simulink model "ES101A_DiagcMgr"  (R2013b)
settings: Solver=ode45  StartTime=0.0  StopTime=0.44  RelTol=1e-3
values from neighbouring files (symbols this model uses):
  BrdgVltg = DataDict.IpSignal    [ES101A_DiagcMgr_DataDict.m]
  DEM_CLEAR_PENDING = DataDict.Constant    [ES101A_DiagcMgr_DataDict.m]
  DEM_DTC_GROUP_ALL_DTCS = DataDict.Constant    [ES101A_DiagcMgr_DataDict.m]
  DFTAGICNTR_CNT_U08 = DataDict.Constant    [ES101A_DiagcMgr_DataDict.m]
  DIAGCMGR_NTCINFOSTSTESTFAILD_CNT_U08 = DataDict.Constant    [ES101A_DiagcMgrProxyX_DataDict.m]    (also in ES101A_DiagcMgr_DataDict.m)
  DIAGCMGR_NTCINFOSTSTESTFAILDTHISIGNCYC_CNT_U08 = DataDict.Constant    [ES101A_DiagcMgr_DataDict.m]
  DIAGCMGR_NTCINFOSTSTESTNOTCMPLTHISIGNCYC_CNT_U08 = DataDict.Constant    [ES101A_DiagcMgrProxyX_DataDict.m]    (also in ES101A_DiagcMgr_DataDict.m)
  DiagcMgrFltResp = DataDict.Calibration    [ES101A_DiagcMgrProxyX_DataDict.m]    (also in ES101A_DiagcMgr_DataDict.m)
  DiagcMgrNtcFltAry = DataDict.NVM    [ES101A_DiagcMgr_DataDict.m]
  DIAGCSTSCTRLDSHTDWNFLTPRSNT_CNT_U16 = DataDict.Constant    [ES101A_DiagcMgr_DataDict.m]
  DIAGCSTSDFTHWAG_CNT_U16 = DataDict.Constant    [ES101A_DiagcMgr_DataDict.m]
  DIAGCSTSDFTHWAGSERLCOMEXPRTVAL_CNT_U16 = DataDict.Constant    [ES101A_DiagcMgr_DataDict.m]
  DIAGCSTSDFTVEHSPD_CNT_U16 = DataDict.Constant    [ES101A_DiagcMgr_DataDict.m]
  DIAGCSTSININVAL_CNT_U16 = DataDict.Constant    [ES101A_DiagcMgrProxyX_DataDict.m]    (also in ES101A_DiagcMgr_DataDict.m)
  DIAGCSTSIVTR1INACTV_CNT_U16 = DataDict.Constant    [ES101A_DiagcMgr_DataDict.m]
  DIAGCSTSIVTR2INACTV_CNT_U16 = DataDict.Constant    [ES101A_DiagcMgr_DataDict.m]
  DIAGCSTSLIMDTPRFMNC_CNT_U16 = DataDict.Constant    [ES101A_DiagcMgr_DataDict.m]
  DIAGCSTSRAMPTOZEROFLTPRSNT_CNT_U16 = DataDict.Constant    [ES101A_DiagcMgr_DataDict.m]
  DIAGCSTSWHLIMBREJCTNDI_CNT_U16 = DataDict.Constant    [ES101A_DiagcMgr_DataDict.m]
  DTCIDXSTSFAIL_CNT_U08 = DataDict.Constant    [ES101A_DiagcMgr_DataDict.m]
  DTCIDXSTSNONTC_CNT_U08 = DataDict.Constant    [ES101A_DiagcMgr_DataDict.m]
  DTCIDXSTSNORES_CNT_U08 = DataDict.Constant    [ES101A_DiagcMgr_DataDict.m]
  DTCIDXSTSPASS_CNT_U08 = DataDict.Constant    [ES101A_DiagcMgr_DataDict.m]
  DTCIDXSTSUPDCFMD_CNT_U08 = DataDict.Constant    [ES101A_DiagcMgr_DataDict.m]
  ELECGLBPRM_IVTRCNT_CNT_U08 = DataDict.ConfigParam    [ES101A_DiagcMgrProxyX_DataDict.m]    (also in ES101A_DiagcMgr_DataDict.m)
  FLTINJ_DIAGCMGR_DIAGCSTSIVTR1INACTV = DataDict.Constant    [ES101A_DiagcMgr_DataDict.m]
  FLTINJ_DIAGCMGR_DIAGCSTSIVTR2INACTV = DataDict.Constant    [ES101A_DiagcMgr_DataDict.m]
  HwTq = DataDict.IpSignal    [ES101A_DiagcMgr_DataDict.m]
  IgnCntr = DataDict.IpSignal    [ES101A_DiagcMgr_DataDict.m]
  MAXDEBCNTRVAL_CNT_S16 = DataDict.Constant    [ES101A_DiagcMgr_DataDict.m]
  MAXRAMPRATE_ULSPERSEC_F32 = DataDict.Constant    [ES101A_DiagcMgrProxyX_DataDict.m]    (also in ES101A_DiagcMgr_DataDict.m)
  MINDEBCNTRVAL_CNT_S16 = DataDict.Constant    [ES101A_DiagcMgr_DataDict.m]
  MINRAMPRATE_ULSPERSEC_F32 = DataDict.Constant    [ES101A_DiagcMgrProxyX_DataDict.m]    (also in ES101A_DiagcMgr_DataDict.m)
  SCAMOTTQCMDTOONE_ULS_F32 = DataDict.Constant    [ES101A_DiagcMgrProxyX_DataDict.m]    (also in ES101A_DiagcMgr_DataDict.m)
  SCAMOTTQCMDTOZERO_ULS_F32 = DataDict.Constant    [ES101A_DiagcMgrProxyX_DataDict.m]    (also in ES101A_DiagcMgr_DataDict.m)
  SysSt = DataDict.IpSignal    [ES101A_DiagcMgr_DataDict.m]
  VehSpd = DataDict.IpSignal    [ES101A_DiagcMgr_DataDict.m]
undefined symbols (not defined in the file or in its folder): ActvMotTqCmdSca, ActvRampRate, AgiCntr, Dem_DTCFormatType, Dem_DTCOriginType, Dem_EventStatusType, DiagcData, DiagcMgrNtcMap, DiagcSts, DtcEnaMask, EcuT, HistNtcFltAry, MicroDiagcData, MotTq, NtcNr, NtcNrWithResd1, NtcStInfo, ProxySetNtcData, Sts, SysSt1, TOTNROFDTC_CNT_U08
libraries: simulink x149, FloatToFixd x5, NxtrNvM x3
(part 10 of 13)

== system ES101A_DiagcMgr/DiagcMgr/SetNtcStsCore/NtcNr is Valid/Diagnostics Not Inhibited/NtcEnabled/NTCSTS_PREFAILD/Update NtcInfoSts, DebCntr and Process RampRate/DebCntr = MAXDEBCNTRVAL_CNT_S16/Update NtcSts and DebCntr ==
  NtcInfo_ArgIn : Inport
  NtcStInfo_ArgIn : Inport  Port=2
  Bus Assignment1 : BusAssignment  AssignedSignals=Sts,NtcStInfo,AgiCntr
  Bus Selector : BusSelector  OutputSignals=Sts,NtcStInfo
  Clear: DIAGCMGR_NTCINFOSTSTESTNOTCMPLTHISIGNCYC_CNT_U08 : Subsystem
  Constant : Constant  Value=MAXDEBCNTRVAL_CNT_S16
  Constant1 : Constant  Value=DIAGCMGR_NTCINFOSTSTESTNOTCMPLTHISIGNCYC_CNT_U08
  Constant2 : Constant  Value=0  OutDataTypeStr=uint8
  Copyright1 : Subsystem  Description=|  mask(Copyright Information){none=on}
      | Copyright info block.                                               
      |                                                                     
      | Place copyright information at the top of every subsystem in design.
      mask prompts: none "No parameters"
      mask help: Place copyright information at the top of every subsystem in design.
      mask Display:
      | NxtrConf = 'Nexteer Confidential';
      | 
      | sys = bdroot; %handle for the current model ("system")
      | first = get_param(sys,'Created');
      | if(isempty(first))
      |     first = datestr(now,'yyyy');
      | else
      |     first = first(end-3:end);  %year is last four digits
      | end
      | 
      | last = get_param(sys,'LastModifiedDate');
      | if isempty(last)
      |     last = datestr(now,'yyyy');
      | else
      |     last = last(end-3:end);
      | end
      | 
      | if strcmp(first,last)
      |     fprintf('%s\nCopyright  %s Nexteer',NxtrConf,first);
      | else
      |     fprintf('%s\n%s%s-%s Nexteer',NxtrConf,char(169),first,last);
      | end
  Set Bit: DIAGCMGR_NTCINFOCFMDNTC_CNT_U08 : simulink/Logic and Bit Operations/Bitwise Operator  logicop=OR  UseBitMask=on  BitMask=DIAGCMGR_NTCINFOCFMDNTC_CNT_U08  BitMaskRealWorld=Stored Integer
  Set Bits: DIAGCMGR_NTCINFOSTSTESTFAILDTHISIGNCYC_CNT_U08 : simulink/Logic and Bit Operations/Bitwise Operator  logicop=OR  UseBitMask=on  BitMask=DIAGCMGR_NTCINFOSTSTESTFAILDTHISIGNCYC_CNT_U08  BitMaskRealWorld=Stored Integer
  Set Bits: DIAGCMGR_NTCINFOSTSTESTFAILD_CNT_U08 : simulink/Logic and Bit Operations/Bitwise Operator  logicop=OR  UseBitMask=on  BitMask=DIAGCMGR_NTCINFOSTSTESTFAILD_CNT_U08  BitMaskRealWorld=Stored Integer
  Update NtcStInfo : simulink/Logic and Bit Operations/Bitwise Operator  logicop=OR  UseBitMask=off  NumInputPorts=2  BitMask=bin2dec('11')  BitMaskRealWorld=Stored Integer
  NtcInfo_ArgOut : Outport
  NtcInfoDebCntr_ArgOut : Outport  Port=2
  wires:
  NtcInfo_ArgIn/1 -> Bus Assignment1/1, Bus Selector/1
  Constant/1 -> NtcInfoDebCntr_ArgOut/1
  Bus Assignment1/1 -> NtcInfo_ArgOut/1
  Clear: DIAGCMGR_NTCINFOSTSTESTNOTCMPLTHISIGNCYC_CNT_U08/1(Out1) -> Bus Assignment1/2
  NtcStInfo_ArgIn/1 -> Update NtcStInfo/2
  Update NtcStInfo/1 -> Bus Assignment1/3
  Bus Selector/2 -> Update NtcStInfo/1  "<NtcStInfo>"
  Constant2/1 -> Bus Assignment1/4
  Constant1/1 -> Clear: DIAGCMGR_NTCINFOSTSTESTNOTCMPLTHISIGNCYC_CNT_U08/2(In1)
  Set Bits: DIAGCMGR_NTCINFOSTSTESTFAILD_CNT_U08/1 -> Set Bits: DIAGCMGR_NTCINFOSTSTESTFAILDTHISIGNCYC_CNT_U08/1
  Set Bits: DIAGCMGR_NTCINFOSTSTESTFAILDTHISIGNCYC_CNT_U08/1 -> Set Bit: DIAGCMGR_NTCINFOCFMDNTC_CNT_U08/1
  Set Bit: DIAGCMGR_NTCINFOCFMDNTC_CNT_U08/1 -> Clear: DIAGCMGR_NTCINFOSTSTESTNOTCMPLTHISIGNCYC_CNT_U08/1(In2)
  Bus Selector/1 -> Set Bits: DIAGCMGR_NTCINFOSTSTESTFAILD_CNT_U08/1  "<Sts>"

== system ES101A_DiagcMgr/DiagcMgr/SetNtcStsCore/NtcNr is Valid/Diagnostics Not Inhibited/NtcEnabled/NTCSTS_PREPASSD/Update NtcInfoSts/Do Nothing/CopyRight2 ==

== system ES101A_DiagcMgr/DiagcMgr/SetNtcStsCore/NtcNr is Valid/Diagnostics Not Inhibited/NtcEnabled/NTCSTS_PREPASSD/Update NtcInfoSts/Update NTC Info's Status Byte & Update the NTC Fault Array/CopyRight2 ==

== system ES101A_DiagcMgr/DiagcMgr/SetNtcStsCore/NtcNr is Valid/Diagnostics Not Inhibited/NtcEnabled/NTCSTS_PREPASSD/Update NtcInfoSts/Update NTC Info's Status Byte & Update the NTC Fault Array/Decrement Counter ==
  "NtcInfo_ArgIn " : Inport
  DebStep_ArgIn : Inport  Port=2
  NtcInfoDebCntr_ArgIn : Inport  Port=3
  Constant : Constant  Value=MINDEBCNTRVAL_CNT_S16
  Copyright1 : Subsystem  Description=|  mask(Copyright Information){none=on}
      | Copyright info block.                                               
      |                                                                     
      | Place copyright information at the top of every subsystem in design.
      mask prompts: none "No parameters"
      mask help: Place copyright information at the top of every subsystem in design.
      mask Display:
      | NxtrConf = 'Nexteer Confidential';
      | 
      | sys = bdroot; %handle for the current model ("system")
      | first = get_param(sys,'Created');
      | if(isempty(first))
      |     first = datestr(now,'yyyy');
      | else
      |     first = first(end-3:end);  %year is last four digits
      | end
      | 
      | last = get_param(sys,'LastModifiedDate');
      | if isempty(last)
      |     last = datestr(now,'yyyy');
      | else
      |     last = last(end-3:end);
      | end
      | 
      | if strcmp(first,last)
      |     fprintf('%s\nCopyright  %s Nexteer',NxtrConf,first);
      | else
      |     fprintf('%s\n%s%s-%s Nexteer',NxtrConf,char(169),first,last);
      | end
  Deb Counter > MINDEBCNTRVAL_CNT_S16 : Subsystem  TreatAsAtomicUnit=on
  DebCntr = MINDEBCNTRVAL_CNT_S16 : Subsystem  TreatAsAtomicUnit=on
  If1 : If  NumInputs=2  IfExpression="u1 <=  u2"
  Merge1 : Merge
  Sub1 : Sum  SaturateOnIntegerOverflow=on
  NtcInfo_ArgOut : Outport
  NtcInfoDebCntr_ArgOut : Outport  Port=2
  wires:
  If1/1 -> DebCntr = MINDEBCNTRVAL_CNT_S16/Action
  If1/2 -> Deb Counter > MINDEBCNTRVAL_CNT_S16/Action
  DebStep_ArgIn/1 -> Sub1/1, Deb Counter > MINDEBCNTRVAL_CNT_S16/1(DebStep)
  "NtcInfo_ArgIn "/1 -> DebCntr = MINDEBCNTRVAL_CNT_S16/1(NtcInfo_ArgIn)
  Constant/1 -> Sub1/2
  Sub1/1 -> If1/2
  Deb Counter > MINDEBCNTRVAL_CNT_S16/1(NtcInfoDebCntr_ArgOut) -> Merge1/2
  DebCntr = MINDEBCNTRVAL_CNT_S16/1(NtcInfo_ArgOut) -> NtcInfo_ArgOut/1
  DebCntr = MINDEBCNTRVAL_CNT_S16/2(NtcInfoDebCntr_ArgOut) -> Merge1/1
  Merge1/1 -> NtcInfoDebCntr_ArgOut/1
  NtcInfoDebCntr_ArgIn/1 -> Deb Counter > MINDEBCNTRVAL_CNT_S16/2(NtcInfoDebCntr_ArgIn), If1/1

== system ES101A_DiagcMgr/DiagcMgr/DiagcMgrPer2/Normal Periodic Processing/For All DTCs/For Each DTC/Check If DTC Status has Changed/DTC Status Changed OR DTC Update NOT Confirmed/Update DTC Status/Dtc Status is Failed/CopyRight2 ==

== system ES101A_DiagcMgr/DiagcMgr/DiagcMgrPer2/Normal Periodic Processing/For All DTCs/For Each DTC/Check If DTC Status has Changed/DTC Status Changed OR DTC Update NOT Confirmed/Update DTC Status/Dtc Status is Failed/Dem_SetEventStatus ==
  EventId : Inport
  EventStatus : Inport  Port=2
  CopyRight2 : Subsystem  Description=|  mask(Copyright Information){none=on}
      | Copyright info block.                                               
      |                                                                     
      | Place copyright information at the top of every subsystem in design.
      mask prompts: none "No parameters"
      mask help: Place copyright information at the top of every subsystem in design.
      mask Display:
      | NxtrConf = 'Nexteer Confidential';
      | 
      | sys = bdroot; %handle for the current model ("system")
      | first = get_param(sys,'Created');
      | first = first(end-3:end);  %year is last four digits
      | 
      | last = get_param(sys,'LastModifiedDate');
      | if isempty(last)
      |     last = datestr(now,'yyyy');
      | else
      |     last = last(end-3:end);
      | end
      | 
      | if strcmp(first,last)
      |     fprintf('%s -- Copyright %s Nexteer',NxtrConf,first)
      | else
      |     fprintf('%s -- %s%s- %s Nexteer',NxtrConf,char(169),first,last)
      | end
  Ground : Ground
  Terminator : Terminator
  Terminator1 : Terminator
  Dem_SetEventStatus_StdRtn : Outport
  wires:
  Ground/1 -> Dem_SetEventStatus_StdRtn/1
  EventStatus/1 -> Terminator1/1
  EventId/1 -> Terminator/1

== system ES101A_DiagcMgr/DiagcMgr/DiagcMgrPer2/Normal Periodic Processing/For All DTCs/For Each DTC/Check If DTC Status has Changed/DTC Status Changed OR DTC Update NOT Confirmed/Update DTC Status/Dtc Status is Failed/Update 'DTC Index Update Confirmed' Bit ==
  Dem_SetEventStatus_StdRtn : Inport
  DtcIdxPrevSts : Inport  Port=2
  DtcIdx : Inport  Port=3
  CopyRight2 : Subsystem  Description=|  mask(Copyright Information){none=on}
      | Copyright info block.                                               
      |                                                                     
      | Place copyright information at the top of every subsystem in design.
      mask prompts: none "No parameters"
      mask help: Place copyright information at the top of every subsystem in design.
      mask Display:
      | NxtrConf = 'Nexteer Confidential';
      | 
      | sys = bdroot; %handle for the current model ("system")
      | first = get_param(sys,'Created');
      | first = first(end-3:end);  %year is last four digits
      | 
      | last = get_param(sys,'LastModifiedDate');
      | if isempty(last)
      |     last = datestr(now,'yyyy');
      | else
      |     last = last(end-3:end);
      | end
      | 
      | if strcmp(first,last)
      |     fprintf('%s -- Copyright %s Nexteer',NxtrConf,first)
      | else
      |     fprintf('%s -- %s%s- %s Nexteer',NxtrConf,char(169),first,last)
      | end
  If : If  IfExpression=u1 == 0  ShowElse=off
  StdRtn is E_OK : Subsystem  TreatAsAtomicUnit=on
  wires:
  DtcIdxPrevSts/1 -> StdRtn is E_OK/2(DtcIdxPrevSts)
  DtcIdx/1 -> StdRtn is E_OK/1(DtcIdx)
  If/1 -> StdRtn is E_OK/Action
  Dem_SetEventStatus_StdRtn/1 -> If/1

== system ES101A_DiagcMgr/DiagcMgr/DiagcMgrPer2/Normal Periodic Processing/For All DTCs/For Each DTC/Check If DTC Status has Changed/DTC Status Changed OR DTC Update NOT Confirmed/Update DTC Status/Dtc Status is No Result or No Ntc/CopyRight2 ==

== system ES101A_DiagcMgr/DiagcMgr/DiagcMgrPer2/Normal Periodic Processing/For All DTCs/For Each DTC/Check If DTC Status has Changed/DTC Status Changed OR DTC Update NOT Confirmed/Update DTC Status/Dtc Status is No Result or No Ntc/Set Bit 7 (DTC Update Confirmed) ==
  In1 : Inport
  Bitwise Operator1 : simulink/Logic and Bit Operations/Bitwise Operator  logicop=OR  UseBitMask=off  NumInputPorts=2  BitMask=bin2dec('11011001')  BitMaskRealWorld=Stored Integer
  CopyRight2 : Subsystem  Description=|  mask(Copyright Information){none=on}
      | Copyright info block.                                               
      |                                                                     
      | Place copyright information at the top of every subsystem in design.
      mask prompts: none "No parameters"
      mask help: Place copyright information at the top of every subsystem in design.
      mask Display:
      | NxtrConf = 'Nexteer Confidential';
      | 
      | sys = bdroot; %handle for the current model ("system")
      | first = get_param(sys,'Created');
      | first = first(end-3:end);  %year is last four digits
      | 
      | last = get_param(sys,'LastModifiedDate');
      | if isempty(last)
      |     last = datestr(now,'yyyy');
      | else
      |     last = last(end-3:end);
      | end
      | 
      | if strcmp(first,last)
      |     fprintf('%s -- Copyright %s Nexteer',NxtrConf,first)
      | else
      |     fprintf('%s -- %s%s- %s Nexteer',NxtrConf,char(169),first,last)
      | end
  DTC Previous Status Bit 7 : Constant  Value=DTCIDXSTSUPDCFMD_CNT_U08
  Out1 : Outport
  wires:
  DTC Previous Status Bit 7/1 -> Bitwise Operator1/2
  In1/1 -> Bitwise Operator1/1
  Bitwise Operator1/1 -> Out1/1

== system ES101A_DiagcMgr/DiagcMgr/DiagcMgrPer2/Normal Periodic Processing/For All DTCs/For Each DTC/Check If DTC Status has Changed/DTC Status Changed OR DTC Update NOT Confirmed/Update DTC Status/Dtc Status is Passed/CopyRight2 ==

== system ES101A_DiagcMgr/DiagcMgr/DiagcMgrPer2/Normal Periodic Processing/For All DTCs/For Each DTC/Check If DTC Status has Changed/DTC Status Changed OR DTC Update NOT Confirmed/Update DTC Status/Dtc Status is Passed/Dem_SetEventStatus ==
  EventId : Inport
  EventStatus : Inport  Port=2
  CopyRight2 : Subsystem  Description=|  mask(Copyright Information){none=on}
      | Copyright info block.                                               
      |                                                                     
      | Place copyright information at the top of every subsystem in design.
      mask prompts: none "No parameters"
      mask help: Place copyright information at the top of every subsystem in design.
      mask Display:
      | NxtrConf = 'Nexteer Confidential';
      | 
      | sys = bdroot; %handle for the current model ("system")
      | first = get_param(sys,'Created');
      | first = first(end-3:end);  %year is last four digits
      | 
      | last = get_param(sys,'LastModifiedDate');
      | if isempty(last)
      |     last = datestr(now,'yyyy');
      | else
      |     last = last(end-3:end);
      | end
      | 
      | if strcmp(first,last)
      |     fprintf('%s -- Copyright %s Nexteer',NxtrConf,first)
      | else
      |     fprintf('%s -- %s%s- %s Nexteer',NxtrConf,char(169),first,last)
      | end
  Ground : Ground
  Terminator : Terminator
  Terminator1 : Terminator
  Dem_SetEventStatus_StdRtn : Outport
  wires:
  EventId/1 -> Terminator/1
  EventStatus/1 -> Terminator1/1
  Ground/1 -> Dem_SetEventStatus_StdRtn/1

== system ES101A_DiagcMgr/DiagcMgr/DiagcMgrPer2/Normal Periodic Processing/For All DTCs/For Each DTC/Check If DTC Status has Changed/DTC Status Changed OR DTC Update NOT Confirmed/Update DTC Status/Dtc Status is Passed/Update 'DTC Index Update Confirmed' Bit ==
  Dem_SetEventStatus_StdRtn : Inport
  DtcIdxPrevSts : Inport  Port=2
  DtcIdx : Inport  Port=3
  CopyRight2 : Subsystem  Description=|  mask(Copyright Information){none=on}
      | Copyright info block.                                               
      |                                                                     
      | Place copyright information at the top of every subsystem in design.
      mask prompts: none "No parameters"
      mask help: Place copyright information at the top of every subsystem in design.
      mask Display:
      | NxtrConf = 'Nexteer Confidential';
      | 
      | sys = bdroot; %handle for the current model ("system")
      | first = get_param(sys,'Created');
      | first = first(end-3:end);  %year is last four digits
      | 
      | last = get_param(sys,'LastModifiedDate');
      | if isempty(last)
      |     last = datestr(now,'yyyy');
      | else
      |     last = last(end-3:end);
      | end
      | 
      | if strcmp(first,last)
      |     fprintf('%s -- Copyright %s Nexteer',NxtrConf,first)
      | else
      |     fprintf('%s -- %s%s- %s Nexteer',NxtrConf,char(169),first,last)
      | end
  If : If  IfExpression=u1 == 0  ShowElse=off
  StdRtn is E_OK : Subsystem  TreatAsAtomicUnit=on
  wires:
  Dem_SetEventStatus_StdRtn/1 -> If/1
  If/1 -> StdRtn is E_OK/Action
  DtcIdx/1 -> StdRtn is E_OK/1(DtcIdx)
  DtcIdxPrevSts/1 -> StdRtn is E_OK/2(DtcIdxPrevSts)

== system ES101A_DiagcMgr/DiagcMgr/SetNtcStsCore/NtcNr is Valid/Diagnostics Not Inhibited/NtcEnabled/NTCSTS_FAILD/Update ISO Bits, Parameter Byte and AgiCntr /ProcessRampResponse and DiagcSts/ControlledShutdown Fault/Atomic Section2 ==
  TmpDiagcSts : Inport
  DiagcData_ArgInOut : Inport  Port=2
  ProxySetNtcData_ArgInOut : Inport  Port=3
  Bitwise Operator : simulink/Logic and Bit Operations/Bitwise Operator  logicop=OR  UseBitMask=off  NumInputPorts=2  BitMask=bin2dec('11011001')  BitMaskRealWorld=Stored Integer
  Bitwise Operator1 : simulink/Logic and Bit Operations/Bitwise Operator  logicop=OR  UseBitMask=off  NumInputPorts=2  BitMask=bin2dec('11011001')  BitMaskRealWorld=Stored Integer
  Bus Creator2 : BusCreator  Inputs=2  OutDataTypeStr=Bus: DiagcData1  NonVirtualBus=on
  Bus Creator3 : BusCreator  Inputs=2  OutDataTypeStr=Bus: DiagcData1  NonVirtualBus=on
  Bus Selector : BusSelector  OutputSignals=DiagcSts,ActvMotTqCmdSca
  Bus Selector1 : BusSelector  OutputSignals=DiagcSts,ActvMotTqCmdSca
  CopyRight2 : Subsystem  Description=|  mask(Copyright Information){none=on}
      | Copyright info block.                                               
      |                                                                     
      | Place copyright information at the top of every subsystem in design.
      mask prompts: none "No parameters"
      mask help: Place copyright information at the top of every subsystem in design.
      mask Display:
      | NxtrConf = 'Nexteer Confidential';
      | 
      | sys = bdroot; %handle for the current model ("system")
      | first = get_param(sys,'Created');
      | first = first(end-3:end);  %year is last four digits
      | 
      | last = get_param(sys,'LastModifiedDate');
      | if isempty(last)
      |     last = datestr(now,'yyyy');
      | else
      |     last = last(end-3:end);
      | end
      | 
      | if strcmp(first,last)
      |     fprintf('%s -- Copyright %s Nexteer',NxtrConf,first)
      | else
      |     fprintf('%s -- %s%s- %s Nexteer',NxtrConf,char(169),first,last)
      | end
  If : If  NumInputs=2  IfExpression=u1 < u2  ShowElse=off
  If3 : If  NumInputs=2  IfExpression=u1 < u2  ShowElse=off
  Scale Motor Torque Command to Zero1 : Constant  Value=SCAMOTTQCMDTOZERO_ULS_F32  OutDataTypeStr=single
  Scale Motor Torque Command to Zero2 : Constant  Value=SCAMOTTQCMDTOZERO_ULS_F32  OutDataTypeStr=single
  Update Scale : Subsystem  TreatAsAtomicUnit=on
  Update Scale1 : Subsystem  TreatAsAtomicUnit=on
  DiagcData_ArgOut : Outport
  ProxySetNtcData_ArgOut : Outport  Port=2
  wires:
  Bus Selector/1 -> Bitwise Operator/1  "<DiagcSts>"
  If/1 -> Update Scale/Action
  Scale Motor Torque Command to Zero1/1 -> If/1
  TmpDiagcSts/1 -> Bitwise Operator1/2, Bitwise Operator/2
  Bus Selector1/1 -> Bitwise Operator1/1  "<DiagcSts>"
  If3/1 -> Update Scale1/Action
  Scale Motor Torque Command to Zero2/1 -> If3/1
  DiagcData_ArgInOut/1 -> Bus Selector/1
  ProxySetNtcData_ArgInOut/1 -> Bus Selector1/1
  Bus Selector/2 -> If/2  "<ActvMotTqCmdSca>"
  Bus Selector1/2 -> If3/2  "<ActvMotTqCmdSca>"
  Bitwise Operator/1 -> Bus Creator2/1
  Update Scale/1(DiagcMgrActvMotTqCmdSca) -> Bus Creator2/2
  Bus Creator2/1 -> DiagcData_ArgOut/1
  Bitwise Operator1/1 -> Bus Creator3/1
  Bus Creator3/1 -> ProxySetNtcData_ArgOut/1
  Update Scale1/1(ProxySetNtcMotTqCmdSca) -> Bus Creator3/2

== system ES101A_DiagcMgr/DiagcMgr/SetNtcStsCore/NtcNr is Valid/Diagnostics Not Inhibited/NtcEnabled/NTCSTS_FAILD/Update ISO Bits, Parameter Byte and AgiCntr /ProcessRampResponse and DiagcSts/ControlledShutdown Fault/CopyRight2 ==

== system ES101A_DiagcMgr/DiagcMgr/SetNtcStsCore/NtcNr is Valid/Diagnostics Not Inhibited/NtcEnabled/NTCSTS_FAILD/Update ISO Bits, Parameter Byte and AgiCntr /ProcessRampResponse and DiagcSts/InformationOnly Fault/Atomic Section2 ==
  DiagcData_ArgInOut : Inport
  ProxySetNtcData_ArgInOut : Inport  Port=2
  TmpDiagcSts : Inport  Port=3
  Bitwise Operator : simulink/Logic and Bit Operations/Bitwise Operator  logicop=OR  UseBitMask=off  NumInputPorts=2  BitMask=bin2dec('11011001')  BitMaskRealWorld=Stored Integer
  Bitwise Operator1 : simulink/Logic and Bit Operations/Bitwise Operator  logicop=OR  UseBitMask=off  NumInputPorts=2  BitMask=bin2dec('11011001')  BitMaskRealWorld=Stored Integer
  Bus Selector : BusSelector  OutputSignals=DiagcSts
  Bus Selector1 : BusSelector  OutputSignals=DiagcSts
  CopyRight2 : Subsystem  Description=|  mask(Copyright Information){none=on}
      | Copyright info block.                                               
      |                                                                     
      | Place copyright information at the top of every subsystem in design.
      mask prompts: none "No parameters"
      mask help: Place copyright information at the top of every subsystem in design.
      mask Display:
      | NxtrConf = 'Nexteer Confidential';
      | 
      | sys = bdroot; %handle for the current model ("system")
      | first = get_param(sys,'Created');
      | first = first(end-3:end);  %year is last four digits
      | 
      | last = get_param(sys,'LastModifiedDate');
      | if isempty(last)
      |     last = datestr(now,'yyyy');
      | else
      |     last = last(end-3:end);
      | end
      | 
      | if strcmp(first,last)
      |     fprintf('%s -- Copyright %s Nexteer',NxtrConf,first)
      | else
      |     fprintf('%s -- %s%s- %s Nexteer',NxtrConf,char(169),first,last)
      | end
  DiagcData_ArgOut : Outport
  ProxySetNtcData_ArgOut : Outport  Port=2
  wires:
  Bus Selector/1 -> Bitwise Operator/1  "<DiagcSts>"
  TmpDiagcSts/1 -> Bitwise Operator1/2, Bitwise Operator/2
  Bus Selector1/1 -> Bitwise Operator1/1  "<DiagcSts>"
  DiagcData_ArgInOut/1 -> Bus Selector/1
  ProxySetNtcData_ArgInOut/1 -> Bus Selector1/1
  Bitwise Operator/1 -> DiagcData_ArgOut/1
  Bitwise Operator1/1 -> ProxySetNtcData_ArgOut/1

== system ES101A_DiagcMgr/DiagcMgr/SetNtcStsCore/NtcNr is Valid/Diagnostics Not Inhibited/NtcEnabled/NTCSTS_FAILD/Update ISO Bits, Parameter Byte and AgiCntr /ProcessRampResponse and DiagcSts/InformationOnly Fault/CopyRight2 ==

== system ES101A_DiagcMgr/DiagcMgr/SetNtcStsCore/NtcNr is Valid/Diagnostics Not Inhibited/NtcEnabled/NTCSTS_FAILD/Update ISO Bits, Parameter Byte and AgiCntr /ProcessRampResponse and DiagcSts/ProcessDiagcSts/CopyRight2 ==

== system ES101A_DiagcMgr/DiagcMgr/SetNtcStsCore/NtcNr is Valid/Diagnostics Not Inhibited/NtcEnabled/NTCSTS_FAILD/Update ISO Bits, Parameter Byte and AgiCntr /ProcessRampResponse and DiagcSts/ProcessDiagcSts/If Action Subsystem ==
  Action Port : ActionPort
  Constant1 : Constant  Value=DIAGCSTSLIMDTPRFMNC_CNT_U16
  Out1 : Outport
  wires:
  Constant1/1 -> Out1/1

== system ES101A_DiagcMgr/DiagcMgr/SetNtcStsCore/NtcNr is Valid/Diagnostics Not Inhibited/NtcEnabled/NTCSTS_FAILD/Update ISO Bits, Parameter Byte and AgiCntr /ProcessRampResponse and DiagcSts/ProcessDiagcSts/If Action Subsystem1 ==
  Action Port : ActionPort
  Constant1 : Constant  Value=0  OutDataTypeStr=uint16
  Out1 : Outport
  wires:
  Constant1/1 -> Out1/1

== system ES101A_DiagcMgr/DiagcMgr/SetNtcStsCore/NtcNr is Valid/Diagnostics Not Inhibited/NtcEnabled/NTCSTS_FAILD/Update ISO Bits, Parameter Byte and AgiCntr /ProcessRampResponse and DiagcSts/ProcessDiagcSts/If Action Subsystem10 ==
  Action Port : ActionPort
  Constant1 : Constant  Value=DIAGCSTSDFTHWAGSERLCOMEXPRTVAL_CNT_U16
  Out1 : Outport
  wires:
  Constant1/1 -> Out1/1

== system ES101A_DiagcMgr/DiagcMgr/SetNtcStsCore/NtcNr is Valid/Diagnostics Not Inhibited/NtcEnabled/NTCSTS_FAILD/Update ISO Bits, Parameter Byte and AgiCntr /ProcessRampResponse and DiagcSts/ProcessDiagcSts/If Action Subsystem11 ==
  Action Port : ActionPort
  Constant1 : Constant  Value=0  OutDataTypeStr=uint16
  Out1 : Outport
  wires:
  Constant1/1 -> Out1/1

== system ES101A_DiagcMgr/DiagcMgr/SetNtcStsCore/NtcNr is Valid/Diagnostics Not Inhibited/NtcEnabled/NTCSTS_FAILD/Update ISO Bits, Parameter Byte and AgiCntr /ProcessRampResponse and DiagcSts/ProcessDiagcSts/If Action Subsystem12 ==
  Action Port : ActionPort
  Constant1 : Constant  Value=DIAGCSTSWHLIMBREJCTNDI_CNT_U16
  Out1 : Outport
  wires:
  Constant1/1 -> Out1/1

== system ES101A_DiagcMgr/DiagcMgr/SetNtcStsCore/NtcNr is Valid/Diagnostics Not Inhibited/NtcEnabled/NTCSTS_FAILD/Update ISO Bits, Parameter Byte and AgiCntr /ProcessRampResponse and DiagcSts/ProcessDiagcSts/If Action Subsystem13 ==
  Action Port : ActionPort
  Constant1 : Constant  Value=0  OutDataTypeStr=uint16
  Out1 : Outport
  wires:
  Constant1/1 -> Out1/1

== system ES101A_DiagcMgr/DiagcMgr/SetNtcStsCore/NtcNr is Valid/Diagnostics Not Inhibited/NtcEnabled/NTCSTS_FAILD/Update ISO Bits, Parameter Byte and AgiCntr /ProcessRampResponse and DiagcSts/ProcessDiagcSts/If Action Subsystem2 ==
  Action Port : ActionPort
  Constant1 : Constant  Value=DIAGCSTSIVTR1INACTV_CNT_U16
  Out1 : Outport
  wires:
  Constant1/1 -> Out1/1

== system ES101A_DiagcMgr/DiagcMgr/SetNtcStsCore/NtcNr is Valid/Diagnostics Not Inhibited/NtcEnabled/NTCSTS_FAILD/Update ISO Bits, Parameter Byte and AgiCntr /ProcessRampResponse and DiagcSts/ProcessDiagcSts/If Action Subsystem3 ==
  Action Port : ActionPort
  Constant1 : Constant  Value=0  OutDataTypeStr=uint16
  Out1 : Outport
  wires:
  Constant1/1 -> Out1/1

== system ES101A_DiagcMgr/DiagcMgr/SetNtcStsCore/NtcNr is Valid/Diagnostics Not Inhibited/NtcEnabled/NTCSTS_FAILD/Update ISO Bits, Parameter Byte and AgiCntr /ProcessRampResponse and DiagcSts/ProcessDiagcSts/If Action Subsystem4 ==
  Action Port : ActionPort
  Constant1 : Constant  Value=DIAGCSTSIVTR2INACTV_CNT_U16
  Out1 : Outport
  wires:
  Constant1/1 -> Out1/1

== system ES101A_DiagcMgr/DiagcMgr/SetNtcStsCore/NtcNr is Valid/Diagnostics Not Inhibited/NtcEnabled/NTCSTS_FAILD/Update ISO Bits, Parameter Byte and AgiCntr /ProcessRampResponse and DiagcSts/ProcessDiagcSts/If Action Subsystem5 ==
  Action Port : ActionPort
  Constant1 : Constant  Value=0  OutDataTypeStr=uint16
  Out1 : Outport
  wires:
  Constant1/1 -> Out1/1

== system ES101A_DiagcMgr/DiagcMgr/SetNtcStsCore/NtcNr is Valid/Diagnostics Not Inhibited/NtcEnabled/NTCSTS_FAILD/Update ISO Bits, Parameter Byte and AgiCntr /ProcessRampResponse and DiagcSts/ProcessDiagcSts/If Action Subsystem6 ==
  Action Port : ActionPort
  Constant1 : Constant  Value=DIAGCSTSDFTHWAG_CNT_U16
  Out1 : Outport
  wires:
  Constant1/1 -> Out1/1

== system ES101A_DiagcMgr/DiagcMgr/SetNtcStsCore/NtcNr is Valid/Diagnostics Not Inhibited/NtcEnabled/NTCSTS_FAILD/Update ISO Bits, Parameter Byte and AgiCntr /ProcessRampResponse and DiagcSts/ProcessDiagcSts/If Action Subsystem7 ==
  Action Port : ActionPort
  Constant1 : Constant  Value=0  OutDataTypeStr=uint16
  Out1 : Outport
  wires:
  Constant1/1 -> Out1/1

== system ES101A_DiagcMgr/DiagcMgr/SetNtcStsCore/NtcNr is Valid/Diagnostics Not Inhibited/NtcEnabled/NTCSTS_FAILD/Update ISO Bits, Parameter Byte and AgiCntr /ProcessRampResponse and DiagcSts/ProcessDiagcSts/If Action Subsystem8 ==
  Action Port : ActionPort
  Constant1 : Constant  Value=DIAGCSTSDFTVEHSPD_CNT_U16
  Out1 : Outport
  wires:
  Constant1/1 -> Out1/1

== system ES101A_DiagcMgr/DiagcMgr/SetNtcStsCore/NtcNr is Valid/Diagnostics Not Inhibited/NtcEnabled/NTCSTS_FAILD/Update ISO Bits, Parameter Byte and AgiCntr /ProcessRampResponse and DiagcSts/ProcessDiagcSts/If Action Subsystem9 ==
  Action Port : ActionPort
  Constant1 : Constant  Value=0  OutDataTypeStr=uint16
  Out1 : Outport
  wires:
  Constant1/1 -> Out1/1

== system ES101A_DiagcMgr/DiagcMgr/SetNtcStsCore/NtcNr is Valid/Diagnostics Not Inhibited/NtcEnabled/NTCSTS_FAILD/Update ISO Bits, Parameter Byte and AgiCntr /ProcessRampResponse and DiagcSts/RapidShutdown Fault/Atomic Section2 ==
  TmpDiagcSts : Inport
  DiagcData_ArgIn : Inport  Port=2
  ProxySetNtcData_ArgIn : Inport  Port=3
  Bitwise Operator2 : simulink/Logic and Bit Operations/Bitwise Operator  logicop=OR  UseBitMask=off  NumInputPorts=2  BitMask=bin2dec('11011001')  BitMaskRealWorld=Stored Integer
  Bitwise Operator3 : simulink/Logic and Bit Operations/Bitwise Operator  logicop=OR  UseBitMask=off  NumInputPorts=2  BitMask=bin2dec('11011001')  BitMaskRealWorld=Stored Integer
  Bus Creator2 : BusCreator  Inputs=3  OutDataTypeStr=Bus: DiagcData1  NonVirtualBus=on
  Bus Creator3 : BusCreator  Inputs=3  OutDataTypeStr=Bus: DiagcData1  NonVirtualBus=on
  Bus Selector1 : BusSelector  OutputSignals=DiagcSts,ActvRampRate,ActvMotTqCmdSca
  Bus Selector2 : BusSelector  OutputSignals=DiagcSts,ActvRampRate,ActvMotTqCmdSca
  CopyRight2 : Subsystem  Description=|  mask(Copyright Information){none=on}
      | Copyright info block.                                               
      |                                                                     
      | Place copyright information at the top of every subsystem in design.
      mask prompts: none "No parameters"
      mask help: Place copyright information at the top of every subsystem in design.
      mask Display:
      | NxtrConf = 'Nexteer Confidential';
      | 
      | sys = bdroot; %handle for the current model ("system")
      | first = get_param(sys,'Created');
      | first = first(end-3:end);  %year is last four digits
      | 
      | last = get_param(sys,'LastModifiedDate');
      | if isempty(last)
      |     last = datestr(now,'yyyy');
      | else
      |     last = last(end-3:end);
      | end
      | 
      | if strcmp(first,last)
      |     fprintf('%s -- Copyright %s Nexteer',NxtrConf,first)
      | else
      |     fprintf('%s -- %s%s- %s Nexteer',NxtrConf,char(169),first,last)
      | end
  If : If  NumInputs=2  IfExpression=u1 > u2  ShowElse=off
  If2 : If  NumInputs=2  IfExpression=u1 > u2  ShowElse=off
  If4 : If  NumInputs=2  IfExpression=u1 < u2  ShowElse=off
  If5 : If  NumInputs=2  IfExpression=u1 < u2  ShowElse=off
  Maximum Ramp Rate : Constant  Value=MAXRAMPRATE_ULSPERSEC_F32  OutDataTypeStr=single
  Maximum Ramp Rate1 : Constant  Value=MAXRAMPRATE_ULSPERSEC_F32  OutDataTypeStr=single
  Scale Motor Torque Command to Zero2 : Constant  Value=SCAMOTTQCMDTOZERO_ULS_F32  OutDataTypeStr=single
  Scale Motor Torque Command to Zero3 : Constant  Value=SCAMOTTQCMDTOZERO_ULS_F32  OutDataTypeStr=single
  Update Ramp Rate : Subsystem  TreatAsAtomicUnit=on
  Update Ramp Rate1 : Subsystem  TreatAsAtomicUnit=on
  Update Scale2 : Subsystem  TreatAsAtomicUnit=on
  Update Scale3 : Subsystem  TreatAsAtomicUnit=on
  "DiagcData_ArgInOut " : Outport
  "ProxySetNtcData_ArgOut " : Outport  Port=2
  wires:
  If/1 -> Update Ramp Rate/Action
  Bus Selector2/3 -> If/2  "<ActvMotTqCmdSca>"
  Maximum Ramp Rate/1 -> If/1
  If2/1 -> Update Ramp Rate1/Action
  Bus Selector1/3 -> If2/2  "<ActvMotTqCmdSca>"
  Maximum Ramp Rate1/1 -> If2/1
  Bus Selector2/1 -> Bitwise Operator2/1  "<DiagcSts>"
  If4/1 -> Update Scale2/Action
  Scale Motor Torque Command to Zero2/1 -> If4/1
  TmpDiagcSts/1 -> Bitwise Operator3/2, Bitwise Operator2/2
  Bus Selector1/1 -> Bitwise Operator3/1  "<DiagcSts>"
  If5/1 -> Update Scale3/Action
  Scale Motor Torque Command to Zero3/1 -> If5/1
  DiagcData_ArgIn/1 -> Bus Selector2/1
  ProxySetNtcData_ArgIn/1 -> Bus Selector1/1
  Bus Selector2/2 -> If4/2  "<ActvRampRate>"
  Bus Selector1/2 -> If5/2  "<ActvRampRate>"
  Bitwise Operator2/1 -> Bus Creator2/1
  Update Scale2/1(DiagcMgrActvMotTqCmdSca) -> Bus Creator2/2
  Bus Creator2/1 -> "DiagcData_ArgInOut "/1
  Bitwise Operator3/1 -> Bus Creator3/1
  Bus Creator3/1 -> "ProxySetNtcData_ArgOut "/1
  Update Scale3/1(ProxySetNtcMotTqCmdSca) -> Bus Creator3/2
  Update Ramp Rate/1(DiagcMgrActvRampRate) -> Bus Creator2/3
  Update Ramp Rate1/1(ProxySetNtcActvRampRate) -> Bus Creator3/3

== system ES101A_DiagcMgr/DiagcMgr/SetNtcStsCore/NtcNr is Valid/Diagnostics Not Inhibited/NtcEnabled/NTCSTS_FAILD/Update ISO Bits, Parameter Byte and AgiCntr /ProcessRampResponse and DiagcSts/RapidShutdown Fault/CopyRight2 ==

== system ES101A_DiagcMgr/DiagcMgr/SetNtcStsCore/NtcNr is Valid/Diagnostics Not Inhibited/NtcEnabled/NTCSTS_FAILD/Update ISO Bits, Parameter Byte and AgiCntr /ProcessRampResponse and DiagcSts/TimedShutdown Fault/Atomic Section2 ==
  TmpDiagcSts : Inport
  RampRate : Inport  Port=2
  DiagcData_ArgIn : Inport  Port=3
  ProxySetNtcData_ArgIn : Inport  Port=4
  Bitwise Operator2 : simulink/Logic and Bit Operations/Bitwise Operator  logicop=OR  UseBitMask=off  NumInputPorts=2  BitMask=bin2dec('11011001')  BitMaskRealWorld=Stored Integer
  Bitwise Operator3 : simulink/Logic and Bit Operations/Bitwise Operator  logicop=OR  UseBitMask=off  NumInputPorts=2  BitMask=bin2dec('11011001')  BitMaskRealWorld=Stored Integer
  Bus Creator2 : BusCreator  Inputs=3  OutDataTypeStr=Bus: DiagcData1  NonVirtualBus=on
  Bus Creator3 : BusCreator  Inputs=3  OutDataTypeStr=Bus: DiagcData1  NonVirtualBus=on
  Bus Selector1 : BusSelector  OutputSignals=DiagcSts,ActvRampRate,ActvMotTqCmdSca
  Bus Selector2 : BusSelector  OutputSignals=DiagcSts,ActvRampRate,ActvMotTqCmdSca
  CopyRight2 : Subsystem  Description=|  mask(Copyright Information){none=on}
      | Copyright info block.                                               
      |                                                                     
      | Place copyright information at the top of every subsystem in design.
      mask prompts: none "No parameters"
      mask help: Place copyright information at the top of every subsystem in design.
      mask Display:
      | NxtrConf = 'Nexteer Confidential';
      | 
      | sys = bdroot; %handle for the current model ("system")
      | first = get_param(sys,'Created');
      | first = first(end-3:end);  %year is last four digits
      | 
      | last = get_param(sys,'LastModifiedDate');
      | if isempty(last)
      |     last = datestr(now,'yyyy');
      | else
      |     last = last(end-3:end);
      | end
      | 
      | if strcmp(first,last)
      |     fprintf('%s -- Copyright %s Nexteer',NxtrConf,first)
      | else
      |     fprintf('%s -- %s%s- %s Nexteer',NxtrConf,char(169),first,last)
      | end
  If : If  NumInputs=2  IfExpression=u1 > u2  ShowElse=off
  If2 : If  NumInputs=2  IfExpression=u1 > u2  ShowElse=off
  If6 : If  NumInputs=2  IfExpression=u1 < u2  ShowElse=off
  If7 : If  NumInputs=2  IfExpression=u1 < u2  ShowElse=off
  Scale Motor Torque Command to Zero3 : Constant  Value=SCAMOTTQCMDTOZERO_ULS_F32  OutDataTypeStr=single
  Scale Motor Torque Command to Zero4 : Constant  Value=SCAMOTTQCMDTOZERO_ULS_F32  OutDataTypeStr=single
  Update Ramp Rate : Subsystem  TreatAsAtomicUnit=on
  Update Ramp Rate1 : Subsystem  TreatAsAtomicUnit=on
  Update Scale2 : Subsystem  TreatAsAtomicUnit=on
  Update Scale3 : Subsystem  TreatAsAtomicUnit=on
  DiagcData_ArgOut : Outport
  ProxySetNtcData_ArgOut : Outport  Port=2
  wires:
  If/1 -> Update Ramp Rate/Action
  Bus Selector2/3 -> If/2  "<ActvMotTqCmdSca>"
  If2/1 -> Update Ramp Rate1/Action
  Bus Selector1/3 -> If2/2  "<ActvMotTqCmdSca>"
  Bus Selector2/1 -> Bitwise Operator2/1  "<DiagcSts>"
  If6/1 -> Update Scale2/Action
  Scale Motor Torque Command to Zero3/1 -> If6/1
  TmpDiagcSts/1 -> Bitwise Operator3/2, Bitwise Operator2/2
  Bus Selector1/1 -> Bitwise Operator3/1  "<DiagcSts>"
  If7/1 -> Update Scale3/Action
  Scale Motor Torque Command to Zero4/1 -> If7/1
  DiagcData_ArgIn/1 -> Bus Selector2/1
  ProxySetNtcData_ArgIn/1 -> Bus Selector1/1
  Bus Selector2/2 -> If6/2  "<ActvRampRate>"
  Bus Selector1/2 -> If7/2  "<ActvRampRate>"
  Bitwise Operator2/1 -> Bus Creator2/1
  Update Scale2/1(DiagcMgrActvMotTqCmdSca) -> Bus Creator2/2
  Bus Creator2/1 -> DiagcData_ArgOut/1
  Bitwise Operator3/1 -> Bus Creator3/1
  Bus Creator3/1 -> ProxySetNtcData_ArgOut/1
  Update Scale3/1(ProxySetNtcMotTqCmdSca) -> Bus Creator3/2
  RampRate/1 -> Update Ramp Rate1/1(RampRate), If2/1, Update Ramp Rate/1(RampRate), If/1
  Update Ramp Rate1/1(ProxySetNtcActvRampRate) -> Bus Creator3/3
  Update Ramp Rate/1(DiagcMgrActvRampRate) -> Bus Creator2/3

== system ES101A_DiagcMgr/DiagcMgr/SetNtcStsCore/NtcNr is Valid/Diagnostics Not Inhibited/NtcEnabled/NTCSTS_FAILD/Update ISO Bits, Parameter Byte and AgiCntr /ProcessRampResponse and DiagcSts/TimedShutdown Fault/CopyRight2 ==

== system ES101A_DiagcMgr/DiagcMgr/SetNtcStsCore/NtcNr is Valid/Diagnostics Not Inhibited/NtcEnabled/NTCSTS_FAILD/Update ISO Bits, Parameter Byte and AgiCntr /UpdSnpshtData/Snapshot Data Enabled/CopyRight2 ==

== system ES101A_DiagcMgr/DiagcMgr/SetNtcStsCore/NtcNr is Valid/Diagnostics Not Inhibited/NtcEnabled/NTCSTS_FAILD/Update ISO Bits, Parameter Byte and AgiCntr /UpdSnpshtData/Snapshot Data Enabled/Initialize ==
  Constant : Constant  OutDataTypeStr=boolean
  Constant1 : Constant  Value=0  OutDataTypeStr=uint8
  CopyRight2 : Subsystem  Description=|  mask(Copyright Information){none=on}
      | Copyright info block.                                               
      |                                                                     
      | Place copyright information at the top of every subsystem in design.
      mask prompts: none "No parameters"
      mask help: Place copyright information at the top of every subsystem in design.
      mask Display:
      | NxtrConf = 'Nexteer Confidential';
      | 
      | sys = bdroot; %handle for the current model ("system")
      | first = get_param(sys,'Created');
      | first = first(end-3:end);  %year is last four digits
      | 
      | last = get_param(sys,'LastModifiedDate');
      | if isempty(last)
      |     last = datestr(now,'yyyy');
      | else
      |     last = last(end-3:end);
      | end
      | 
      | if strcmp(first,last)
      |     fprintf('%s -- Copyright %s Nexteer',NxtrConf,first)
      | else
      |     fprintf('%s -- %s%s- %s Nexteer',NxtrConf,char(169),first,last)
      | end
  Data Store Write : DataStoreWrite  DataStoreName=SnpshtDataAryIdxInvld
  Data Store Write1 : DataStoreWrite  DataStoreName=SnpshtDataAryIdx
  wires:
  Constant1/1 -> Data Store Write1/1
  Constant/1 -> Data Store Write/1

== system ES101A_DiagcMgr/DiagcMgr/SetNtcStsCore/NtcNr is Valid/Diagnostics Not Inhibited/NtcEnabled/NTCSTS_FAILD/Update ISO Bits, Parameter Byte and AgiCntr /UpdSnpshtData/Snapshot Data Enabled/While  ==
  NtcNr : Inport
  NtcStInfo : Inport  Port=2
  SnapshotDataBus : Inport  Port=3
  CopyRight2 : Subsystem  Description=|  mask(Copyright Information){none=on}
      | Copyright info block.                                               
      |                                                                     
      | Place copyright information at the top of every subsystem in design.
      mask prompts: none "No parameters"
      mask help: Place copyright information at the top of every subsystem in design.
      mask Display:
      | NxtrConf = 'Nexteer Confidential';
      | 
      | sys = bdroot; %handle for the current model ("system")
      | first = get_param(sys,'Created');
      | first = first(end-3:end);  %year is last four digits
      | 
      | last = get_param(sys,'LastModifiedDate');
      | if isempty(last)
      |     last = datestr(now,'yyyy');
      | else
      |     last = last(end-3:end);
      | end
      | 
      | if strcmp(first,last)
      |     fprintf('%s -- Copyright %s Nexteer',NxtrConf,first)
      | else
      |     fprintf('%s -- %s%s- %s Nexteer',NxtrConf,char(169),first,last)
      | end
  Logical Operator : Logic  AllPortsSameDT=off  OutDataTypeStr=boolean
  Relational Operator : RelationalOperator  Operator=<  OutDataTypeStr=boolean
  Snapshot Data Array : DataStoreRead  DataStoreName=SnpShtDataAry
  Snapshot Data Array Index : DataStoreRead  DataStoreName=SnpshtDataAryIdx
  Snapshot Data Array Index Invalid : DataStoreRead  DataStoreName=SnpshtDataAryIdxInvld
  While Iterator Subsystem : Subsystem  Priority=2  TreatAsAtomicUnit=on
      settings: AttributesFormatString=Priority = %<Priority>
  Width : Width
  wires:
  Width/1 -> Relational Operator/2
  Logical Operator/1 -> While Iterator Subsystem/2(cond), While Iterator Subsystem/1(IC)
  Snapshot Data Array Index Invalid/1 -> Logical Operator/1
  Relational Operator/1 -> Logical Operator/2
  Snapshot Data Array Index/1 -> Relational Operator/1
  Snapshot Data Array/1 -> Width/1
  SnapshotDataBus/1 -> While Iterator Subsystem/5(SnapshotDataBus)
  NtcStInfo/1 -> While Iterator Subsystem/4(NtcStInfo)
  NtcNr/1 -> While Iterator Subsystem/3(NtcNr)

== system ES101A_DiagcMgr/DiagcMgr/SetNtcStsCore/NtcNr is Valid/Diagnostics Not Inhibited/NtcEnabled/NTCSTS_PREFAILD/Update NtcInfoSts, DebCntr and Process RampRate/Deb Counter < MAXDEBCNTRVAL_CNT_S16/DebCntr = DebCntr + DebStep/Copyright1 ==

== system ES101A_DiagcMgr/DiagcMgr/SetNtcStsCore/NtcNr is Valid/Diagnostics Not Inhibited/NtcEnabled/NTCSTS_PREFAILD/Update NtcInfoSts, DebCntr and Process RampRate/Deb Counter < MAXDEBCNTRVAL_CNT_S16/DebCntr = DebStep/Copyright1 ==

== system ES101A_DiagcMgr/DiagcMgr/SetNtcStsCore/NtcNr is Valid/Diagnostics Not Inhibited/NtcEnabled/NTCSTS_PREFAILD/Update NtcInfoSts, DebCntr and Process RampRate/DebCntr = MAXDEBCNTRVAL_CNT_S16/ProcessRampResponse and DiagcSts/ControlledShutdown Fault ==
  DiagcData_ArgInOut : Inport
  ProxySetNtcData_ArgInOut : Inport  Port=2
  TmpDiagcSts : Inport  Port=3
  Action Port : ActionPort
  Atomic Section2 : Subsystem  Description=|  RequirementInfo="{'linktype_rmi_doors' '0000c474 (/ESG Group/FDD Module Requirements/EA4 Specific/ES101A_DiagcMgr)' '#ES101A_300' 'true' 'REQ:  ES101A_300' '' } %GIDa_d5604592_eee3_49e3_8114_6c2b4a501bb3"
      | EXCLUSIVE AREA:
      | Write data into the DiagcSts Register & ActvRampRate Register
      settings: AttributesFormatString=%<Description>
  Bitwise Operator : simulink/Logic and Bit Operations/Bitwise Operator  logicop=OR  UseBitMask=off  NumInputPorts=3  BitMask=bin2dec('11011001')  BitMaskRealWorld=Stored Integer
  CopyRight2 : Subsystem  Description=|  mask(Copyright Information){none=on}
      | Copyright info block.                                               
      |                                                                     
      | Place copyright information at the top of every subsystem in design.
      mask prompts: none "No parameters"
      mask help: Place copyright information at the top of every subsystem in design.
      mask Display:
      | NxtrConf = 'Nexteer Confidential';
      | 
      | sys = bdroot; %handle for the current model ("system")
      | first = get_param(sys,'Created');
      | first = first(end-3:end);  %year is last four digits
      | 
      | last = get_param(sys,'LastModifiedDate');
      | if isempty(last)
      |     last = datestr(now,'yyyy');
      | else
      |     last = last(end-3:end);
      | end
      | 
      | if strcmp(first,last)
      |     fprintf('%s -- Copyright %s Nexteer',NxtrConf,first)
      | else
      |     fprintf('%s -- %s%s- %s Nexteer',NxtrConf,char(169),first,last)
      | end
  Diagnostic Status Controlled Shutdown Fault Present : Constant  Value=DIAGCSTSCTRLDSHTDWNFLTPRSNT_CNT_U16
  Ramp To Zero Fault Present : Constant  Value=DIAGCSTSRAMPTOZEROFLTPRSNT_CNT_U16  OutDataTypeStr=uint16
  DiagcData_ArgOut : Outport
  ProxySetNtcData_ArgOut : Outport  Port=2
  wires:
  Diagnostic Status Controlled Shutdown Fault Present/1 -> Bitwise Operator/1
  Ramp To Zero Fault Present/1 -> Bitwise Operator/2
  Bitwise Operator/1 -> Atomic Section2/1(TmpDiagcSts)
  TmpDiagcSts/1 -> Bitwise Operator/3
  DiagcData_ArgInOut/1 -> Atomic Section2/2(DiagcData_ArgInOut)
  ProxySetNtcData_ArgInOut/1 -> Atomic Section2/3(ProxySetNtcData_ArgInOut)
  Atomic Section2/1(DiagcData_ArgOut) -> DiagcData_ArgOut/1
  Atomic Section2/2(ProxySetNtcData_ArgOut) -> ProxySetNtcData_ArgOut/1

== system ES101A_DiagcMgr/DiagcMgr/SetNtcStsCore/NtcNr is Valid/Diagnostics Not Inhibited/NtcEnabled/NTCSTS_PREFAILD/Update NtcInfoSts, DebCntr and Process RampRate/DebCntr = MAXDEBCNTRVAL_CNT_S16/ProcessRampResponse and DiagcSts/CopyRight2 ==

== system ES101A_DiagcMgr/DiagcMgr/SetNtcStsCore/NtcNr is Valid/Diagnostics Not Inhibited/NtcEnabled/NTCSTS_PREFAILD/Update NtcInfoSts, DebCntr and Process RampRate/DebCntr = MAXDEBCNTRVAL_CNT_S16/ProcessRampResponse and DiagcSts/InformationOnly Fault ==
  DiagcData_ArgIn : Inport
  ProxySetNtcData_ArgIn : Inport  Port=2
  TmpDiagcSts : Inport  Port=3
  Action Port : ActionPort
  Atomic Section2 : Subsystem  Description=|  RequirementInfo="{'linktype_rmi_doors' '0000c474 (/ESG Group/FDD Module Requirements/EA4 Specific/ES101A_DiagcMgr)' '#ES101A_300' 'true' 'REQ:  ES101A_300' '' } %GIDa_3a29d3e2_9b31_44fb_8987_05525ef511dc"
      | EXCLUSIVE AREA:
      | Write data into the DiagcSts Register & ActvRampRate Register
      settings: AttributesFormatString=%<Description>
  CopyRight2 : Subsystem  Description=|  mask(Copyright Information){none=on}
      | Copyright info block.                                               
      |                                                                     
      | Place copyright information at the top of every subsystem in design.
      mask prompts: none "No parameters"
      mask help: Place copyright information at the top of every subsystem in design.
      mask Display:
      | NxtrConf = 'Nexteer Confidential';
      | 
      | sys = bdroot; %handle for the current model ("system")
      | first = get_param(sys,'Created');
      | first = first(end-3:end);  %year is last four digits
      | 
      | last = get_param(sys,'LastModifiedDate');
      | if isempty(last)
      |     last = datestr(now,'yyyy');
      | else
      |     last = last(end-3:end);
      | end
      | 
      | if strcmp(first,last)
      |     fprintf('%s -- Copyright %s Nexteer',NxtrConf,first)
      | else
      |     fprintf('%s -- %s%s- %s Nexteer',NxtrConf,char(169),first,last)
      | end
  DiagcData_ArgOut : Outport
  ProxySetNtcData_ArgOut : Outport  Port=2
  wires:
  DiagcData_ArgIn/1 -> Atomic Section2/1(DiagcData_ArgInOut)
  ProxySetNtcData_ArgIn/1 -> Atomic Section2/2(ProxySetNtcData_ArgInOut)
  Atomic Section2/1(DiagcData_ArgOut) -> DiagcData_ArgOut/1
  Atomic Section2/2(ProxySetNtcData_ArgOut) -> ProxySetNtcData_ArgOut/1
  TmpDiagcSts/1 -> Atomic Section2/3(TmpDiagcSts)
